simulink subsystem "PvtSubSys_VSM_LCK"  (R2020b)
settings: Solver=VariableStepAuto  StartTime=0.0  StopTime=10.0  RelTol=1e-3
values from neighbouring files (symbols this model uses):
  LCK_STATE : value not decoded    [LCK.sldd]
  P_VSM_LCK_A1 = 15.0    [LCK.sldd]
  P_VSM_LCK_AbsEspInTime = 3.0    [LCK.sldd]
  P_VSM_LCK_absLongitudeAccIn = 2.5    [LCK.sldd]
  P_VSM_LCK_absLongitudeAccOut = 3.0    [LCK.sldd]
  P_VSM_LCK_AccRateIn = 30.0    [LCK.sldd]
  P_VSM_LCK_AccRateInTime = 1.5    [LCK.sldd]
  P_VSM_LCK_AccRateOut = 80.0    [LCK.sldd]
  P_VSM_LCK_AccrPelOut = 30.0    [LCK.sldd]
  P_VSM_LCK_AccrPelRateOut = 0.0    [LCK.sldd]
  P_VSM_LCK_BrakePressIn = 3.0    [LCK.sldd]
  P_VSM_LCK_BrakePressInTime = 1.5    [LCK.sldd]
  P_VSM_LCK_BrakePressOut = 5.0    [LCK.sldd]
  P_VSM_LCK_C0 = 0.4    [LCK.sldd]
  P_VSM_LCK_DrvInputTrqValueIn = 2.0    [LCK.sldd]
  P_VSM_LCK_DrvInputTrqValueInTime = 3.0    [LCK.sldd]
  P_VSM_LCK_DrvInputTrqValueOut = 2.3    [LCK.sldd]
  P_VSM_LCK_dypreFactor = 1.0    [LCK.sldd]
  P_VSM_LCK_IdleInTime = 2.0    [LCK.sldd]
  P_VSM_LCK_LanechangeSwitch = 0.0    [LCK.sldd]
  P_VSM_LCK_LaneDouble = 1.0    [LCK.sldd]
  P_VSM_LCK_Lanewidthswitch = 1.0    [LCK.sldd]
  P_VSM_LCK_LateralAcceIn = 3.0    [LCK.sldd]
  P_VSM_LCK_LateralAcceInTime = 3.0    [LCK.sldd]
  P_VSM_LCK_LateralAcceOut = 3.5    [LCK.sldd]
  P_VSM_LCK_LCDrvInputTrqValueOut = 3.0    [LCK.sldd]
  P_VSM_LCK_LCOverrideTime = 0.6    [LCK.sldd]
  P_VSM_LCK_LCOverrideValue = 1.5    [LCK.sldd]
  P_VSM_LCK_LongitudeAccIn = 3.0    [LCK.sldd]
  P_VSM_LCK_LongitudeAccInTime = 3.0    [LCK.sldd]
  P_VSM_LCK_LongitudeAccOut = 3.5    [LCK.sldd]
  P_VSM_LCK_OverrideInTime = 3.0    [LCK.sldd]
  P_VSM_LCK_OverrideTime = 0.3    [LCK.sldd]
  P_VSM_LCK_OverrideValue = 1.2    [LCK.sldd]
  P_VSM_LCK_ParamA1 : value not decoded    [LCK.sldd]
  P_VSM_LCK_PreTime = 0.2    [LCK.sldd]
  P_VSM_LCK_State_Absesp_enable = 1.0    [LCK.sldd]
  P_VSM_LCK_State_Accpedalrate_enable = 0.0    [LCK.sldd]
  P_VSM_LCK_State_Breakpressure_enable = 1.0    [LCK.sldd]
  P_VSM_LCK_State_DriverInputTrqValue_enable = 1.0    [LCK.sldd]
  P_VSM_LCK_State_Eps_enable = 1.0    [LCK.sldd]
  P_VSM_LCK_State_ESSSts_enable = 1.0    [LCK.sldd]
  P_VSM_LCK_State_GEAR_enable = 1.0    [LCK.sldd]
  P_VSM_LCK_State_Handson_enable = 1.0    [LCK.sldd]
  P_VSM_LCK_State_IdleInTime_enable = 0.0    [LCK.sldd]
  P_VSM_LCK_State_Lane_enable = 1.0    [LCK.sldd]
  P_VSM_LCK_State_LaneChange_enable = 1.0    [LCK.sldd]
  P_VSM_LCK_State_LaneCurve_enable = 0.0    [LCK.sldd]
  P_VSM_LCK_State_LateralAcce_enable = 1.0    [LCK.sldd]
  P_VSM_LCK_State_LongitudeAcc_enable = 1.0    [LCK.sldd]
  P_VSM_LCK_State_LSMLine_enable = 1.0    [LCK.sldd]
  P_VSM_LCK_State_Overide_enable = 1.0    [LCK.sldd]
  P_VSM_LCK_State_Param_LaneCurve : value not decoded    [LCK.sldd]
  P_VSM_LCK_State_Param_LaneCurve_Offset : value not decoded    [LCK.sldd]
  P_VSM_LCK_State_Param_LaneWidth : value not decoded    [LCK.sldd]
  P_VSM_LCK_State_Param_LaneWidth_Offset : value not decoded    [LCK.sldd]
  P_VSM_LCK_State_SteerWheelAngle_enable = 1.0    [LCK.sldd]
  P_VSM_LCK_State_SteerWheelSpd_enable = 1.0    [LCK.sldd]
  P_VSM_LCK_State_TargetLaneIn_enable = 1.0    [LCK.sldd]
  P_VSM_LCK_State_TurnLight_enable = 1.0    [LCK.sldd]
  P_VSM_LCK_State_Vehspeed_enable = 1.0    [LCK.sldd]
  P_VSM_LCK_State_Yawsup_enable = 1.0    [LCK.sldd]
  P_VSM_LCK_SteerAngleSpdIn = 150.0    [LCK.sldd]
  P_VSM_LCK_SteerAngleSpdInTime = 3.0    [LCK.sldd]
  P_VSM_LCK_SteerAngleSpdOut = 200.0    [LCK.sldd]
  P_VSM_LCK_SteerWheelAngleIn = 70.0    [LCK.sldd]
  P_VSM_LCK_SteerWheelAngleInTime = 3.0    [LCK.sldd]
  P_VSM_LCK_SteerWheelAngleOut = 90.0    [LCK.sldd]
  P_VSM_LCK_T0 = 0.75    [LCK.sldd]
  P_VSM_LCK_T1 = 15.0    [LCK.sldd]
  P_VSM_LCK_TargetInSwitch = 0.0    [LCK.sldd]
  P_VSM_LCK_Warnarea1 = -0.55    [LCK.sldd]
  P_VSM_LCK_Warnarea2 = -0.35    [LCK.sldd]
  P_VSM_LCK_YawRateIn = 0.2    [LCK.sldd]
  P_VSM_LCK_YawRateInTime = 1.0    [LCK.sldd]
  P_VSM_LCK_YawRateOut = 0.25    [LCK.sldd]
undefined symbols (not defined in the file or in its folder): P_VSM_LSMC_SampleTime
libraries: simulink x275
(part 3 of 5)

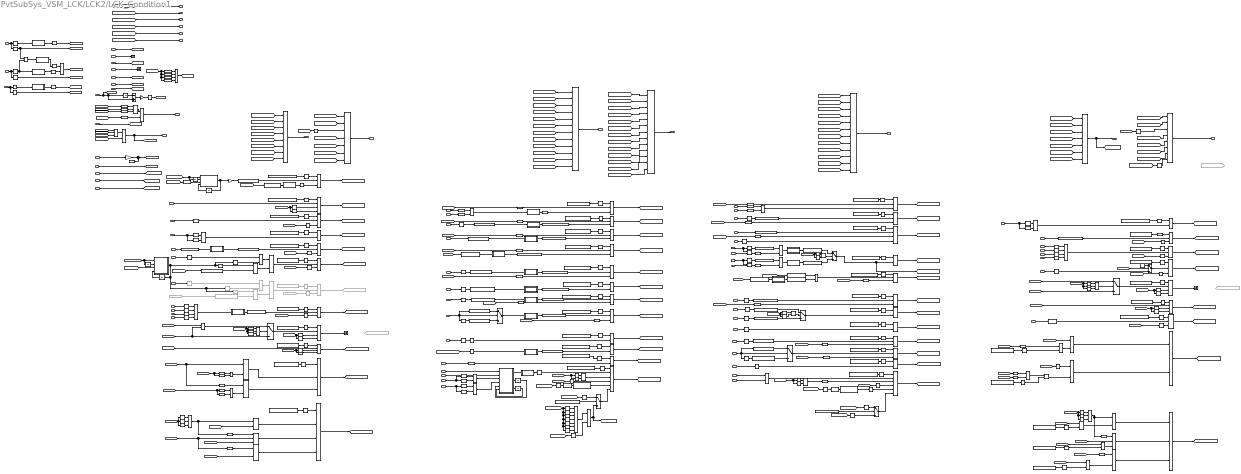
== system PvtSubSys_VSM_LCK/LCK2/LCK_Condition1 ==
  note: 2,3=wrong
  note: Idle2Ready
  note: other2Idle
  note: Active2Ready
  note: Ready2Active
  note: LCK修改记录202010/21
      | 1、去掉TJAlinevalid/LCKlinevalid ;
      |
      |
      |
      |
      | 注：HWAActive=true；将抑制
      | （1）转向灯条件
      | （2）刹车信号；
      | （3）加速踏板信号；
      |
      | 20201102:
      |   TargetP0Exit 换为 TJALineValid
  TJAOn : Inport
  TJASts : Inport  Port=2
  HWAACTIVE : Inport  Port=3
  LCKOn : Inport  Port=4
  VehicleSpd : Inport  Port=5
  VehicleYawRate_rads : Inport  Port=6
  LeftTurnSw : Inport  Port=7
  RightTurnSw : Inport  Port=8
  ECMAccrPellPosnDiagc : Inport  Port=9
  SteerAngleSpd : Inport  Port=10
  ESP_MasterCylindBrakePress : Inport  Port=11
  EPS_DrvInputTrqValue : Inport  Port=12
  EPS_LKATrqOvlDlvdSts : Inport  Port=13
  LKATrqOvlCmdReqValue : Inport  Port=14
  LCKSts : Inport  Port=15
  canESPVDCActive : Inport  Port=16
  canESPPTCActive : Inport  Port=17
  canESPBTCActive : Inport  Port=18
  canABSABSActive : Inport  Port=19
  HandsOffWarnLevel : Inport  Port=20
  canSASSteerWheelAngle : Inport  Port=21
  canABMLateralAcce : Inport  Port=22
  LongitudeAcc : Inport  Port=23
  HandsOn : Inport  Port=24
  TJALineValid : Inport  Port=25
  CURRENT_GEAR : Inport  Port=26
  ESSSts : Inport  Port=27
  LaneCurve : Inport  Port=28
  HWASts : Inport  Port=29
  TJALCKState : Inport  Port=30
  LSSSwtReq : Inport  Port=31
  LeftChange : Inport  Port=32
  RightChange : Inport  Port=33
  FLWhelDy : Inport  Port=34
  FRWhelDy : Inport  Port=35
  LCK_TargetLaneIn : Inport  Port=36
  LCKLineValid : Inport  Port=37
  HWALineValid : Inport  Port=38
  VehConfigLCK : Inport  Port=39
  PLAN_ALC_stsReason : Inport  Port=40
  NOH_Sts : Inport  Port=41
  LSM_PilotRoadSts : Inport  Port=42
  BrkPedalSts : Inport  Port=43
  Abs{,1..10,14..16} (14 alike) : Abs
  Add : Sum  Inputs=-+
  CURRENT_GEAR2 : InportShadow  Port=26
  Compare To Constant : simulink/Logic and Bit Operations/Compare To Constant  relop=<=  const=55  OutDataTypeStr=boolean
  Compare To Constant1 : simulink/Logic and Bit Operations/Compare To Constant  relop=>=  const=P_VSM_LCK_YawRateOut  OutDataTypeStr=boolean
  Compare To Constant10 : simulink/Logic and Bit Operations/Compare To Constant  relop=>  const=0.5  OutDataTypeStr=boolean
  Compare To Constant{100..101,113,125,250} (5 alike) : simulink/Logic and Bit Operations/Compare To Constant  relop===  const=3  OutDataTypeStr=boolean
  Compare To Constant102 : simulink/Logic and Bit Operations/Compare To Constant  relop===  const=2  OutDataTypeStr=boolean
  Compare To Constant103 : simulink/Logic and Bit Operations/Compare To Constant  relop===  const=2  OutDataTypeStr=boolean
  Compare To Constant{2,4..5,14,17,24,33,36,38,48,51,59,63,66,68,70,72,77,81,85,104..105,107,114,116..118,120,124,127..128,157,165,171,173,176,179,181..182,186,188,195..197,199,207,211..212,226..227,229..231,242,245,248} (56 alike) : simulink/Logic and Bit Operations/Compare To Constant  relop===  const=0  OutDataTypeStr=boolean
  Compare To Constant{6,12,15..16,18,20..22,37,39,44,46,56,67,71,74..75,82..83,86,88,90,94,96,106,119,145,166..167,169..170,172,174..175,184,187,193..194,205,208..209,233..234,240,243,246} (46 alike) : simulink/Logic and Bit Operations/Compare To Constant  relop===  const=1  OutDataTypeStr=boolean
  Compare To Constant108 : simulink/Logic and Bit Operations/Compare To Constant  relop=>=  const=3  OutDataTypeStr=boolean
  Compare To Constant109 : simulink/Logic and Bit Operations/Compare To Constant  relop=<=  const=2  OutDataTypeStr=boolean
  Compare To Constant11 : simulink/Logic and Bit Operations/Compare To Constant  relop===  const=8  OutDataTypeStr=boolean
  Compare To Constant110 : simulink/Logic and Bit Operations/Compare To Constant  relop===  const=8  OutDataTypeStr=boolean
  Compare To Constant111 : simulink/Logic and Bit Operations/Compare To Constant  relop===  const=LCK_STATE.LCK_Idle  OutDataTypeStr=boolean
  Compare To Constant112 : simulink/Logic and Bit Operations/Compare To Constant  relop===  const=10  OutDataTypeStr=boolean
  Compare To Constant115 : simulink/Logic and Bit Operations/Compare To Constant  relop===  const=9  OutDataTypeStr=boolean
  Compare To Constant121 : simulink/Logic and Bit Operations/Compare To Constant  relop=<  const=P_VSM_LCK_AccRateIn  OutDataTypeStr=boolean
  Compare To Constant123 : simulink/Logic and Bit Operations/Compare To Constant  relop=<  const=P_VSM_LCK_SteerWheelAngleIn  OutDataTypeStr=boolean
  Compare To Constant126 : simulink/Logic and Bit Operations/Compare To Constant  relop===  const=9  OutDataTypeStr=boolean
  Compare To Constant129 : simulink/Logic and Bit Operations/Compare To Constant  relop=<  const=P_VSM_LCK_LateralAcceIn  OutDataTypeStr=boolean
  Compare To Constant13 : simulink/Logic and Bit Operations/Compare To Constant  relop=<  const=P_VSM_LCK_DrvInputTrqValueIn  OutDataTypeStr=boolean
  Compare To Constant130 : simulink/Logic and Bit Operations/Compare To Constant  relop=<  const=P_VSM_LCK_LongitudeAccIn  OutDataTypeStr=boolean
  Compare To Constant131 : simulink/Logic and Bit Operations/Compare To Constant  relop=<  const=P_VSM_LCK_absLongitudeAccIn  OutDataTypeStr=boolean
  Compare To Constant132 : simulink/Logic and Bit Operations/Compare To Constant  relop===  const=19  OutDataTypeStr=boolean
  Compare To Constant133 : simulink/Logic and Bit Operations/Compare To Constant  relop===  const=20  OutDataTypeStr=boolean
  Compare To Constant134 : simulink/Logic and Bit Operations/Compare To Constant  relop===  const=25  OutDataTypeStr=boolean
  Compare To Constant135 : simulink/Logic and Bit Operations/Compare To Constant  Commented=on  relop===  const=0  OutDataTypeStr=boolean
  Compare To Constant136 : simulink/Logic and Bit Operations/Compare To Constant  relop=>=  const=P_VSM_LCK_AccrPelRateOut  OutDataTypeStr=boolean
  Compare To Constant137 : simulink/Logic and Bit Operations/Compare To Constant  Commented=on  relop===  const=1  OutDataTypeStr=boolean
  Compare To Constant138 : simulink/Logic and Bit Operations/Compare To Constant  Commented=on  relop===  const=0  OutDataTypeStr=boolean
  Compare To Constant{35,41,54,78,80,139,164,177,238,256,258} (11 alike) : simulink/Logic and Bit Operations/Compare To Constant  relop===  const=5  OutDataTypeStr=boolean
  Compare To Constant140 : simulink/Logic and Bit Operations/Compare To Constant  Commented=on  relop===  const=LCK_STATE.LCK_Idle  OutDataTypeStr=boolean
  Compare To Constant141 : simulink/Logic and Bit Operations/Compare To Constant  Commented=on  relop===  const=1  OutDataTypeStr=boolean
  Compare To Constant142 : simulink/Logic and Bit Operations/Compare To Constant  relop===  const=26  OutDataTypeStr=boolean
  Compare To Constant143 : simulink/Logic and Bit Operations/Compare To Constant  relop===  const=30  OutDataTypeStr=boolean
  Compare To Constant144 : simulink/Logic and Bit Operations/Compare To Constant  relop=>=  const=3  OutDataTypeStr=boolean
  Compare To Constant146 : simulink/Logic and Bit Operations/Compare To Constant  relop=<  const=150  OutDataTypeStr=boolean
  Compare To Constant147 : simulink/Logic and Bit Operations/Compare To Constant  relop=>  const=155  OutDataTypeStr=boolean
  Compare To Constant{69,79,150,153,158,163,178,210,239,251,257,259} (12 alike) : simulink/Logic and Bit Operations/Compare To Constant  relop===  const=6  OutDataTypeStr=boolean
  Compare To Constant159 : simulink/Logic and Bit Operations/Compare To Constant  relop=~=  const=5  OutDataTypeStr=boolean
  Compare To Constant160 : simulink/Logic and Bit Operations/Compare To Constant  relop=~=  const=6  OutDataTypeStr=boolean
  Compare To Constant161 : simulink/Logic and Bit Operations/Compare To Constant  relop=~=  const=5  OutDataTypeStr=boolean
  Compare To Constant162 : simulink/Logic and Bit Operations/Compare To Constant  relop=~=  const=6  OutDataTypeStr=boolean
  Compare To Constant19 : simulink/Logic and Bit Operations/Compare To Constant  relop=>=  const=55  OutDataTypeStr=boolean
  Compare To Constant213 : simulink/Logic and Bit Operations/Compare To Constant  relop=<  const=0  OutDataTypeStr=boolean
  Compare To Constant214 : simulink/Logic and Bit Operations/Compare To Constant  relop=>  const=P_VSM_LCK_LCOverrideValue  OutDataTypeStr=boolean
  Compare To Constant228 : simulink/Logic and Bit Operations/Compare To Constant  relop=>=  const=P_VSM_LCK_IdleInTime  OutDataTypeStr=boolean
  Compare To Constant235 : simulink/Logic and Bit Operations/Compare To Constant  Commented=on  relop===  const=1  OutDataTypeStr=boolean
  Compare To Constant237 : simulink/Logic and Bit Operations/Compare To Constant  relop=>  const=P_VSM_LCK_LCOverrideTime  OutDataTypeStr=boolean
  Compare To Constant{8,42,241,244,247} (5 alike) : simulink/Logic and Bit Operations/Compare To Constant  relop=>  const=3  OutDataTypeStr=boolean
  Compare To Constant249 : simulink/Logic and Bit Operations/Compare To Constant  relop=>  const=P_VSM_LCK_LCDrvInputTrqValueOut  OutDataTypeStr=boolean
  Compare To Constant25 : simulink/Logic and Bit Operations/Compare To Constant  relop=<  const=P_VSM_LCK_BrakePressIn  OutDataTypeStr=boolean
  Compare To Constant252 : simulink/Logic and Bit Operations/Compare To Constant  relop===  const=9  OutDataTypeStr=boolean
  Compare To Constant253 : simulink/Logic and Bit Operations/Compare To Constant  relop===  const=10  OutDataTypeStr=boolean
  Compare To Constant27 : simulink/Logic and Bit Operations/Compare To Constant  relop=>  const=P_VSM_LCK_BrakePressOut  OutDataTypeStr=boolean
  Compare To Constant29 : simulink/Logic and Bit Operations/Compare To Constant  relop=<  const=P_VSM_LCK_YawRateIn  OutDataTypeStr=boolean
  Compare To Constant3 : simulink/Logic and Bit Operations/Compare To Constant  relop===  const=8  OutDataTypeStr=boolean
  Compare To Constant34 : simulink/Logic and Bit Operations/Compare To Constant  relop=<  const=0.005  OutDataTypeStr=boolean
  Compare To Constant40 : simulink/Logic and Bit Operations/Compare To Constant  relop=>=  const=P_VSM_LCK_AccrPelOut  OutDataTypeStr=boolean
  Compare To Constant43 : simulink/Logic and Bit Operations/Compare To Constant  relop===  const=LCK_STATE.LCK_Idle  OutDataTypeStr=boolean
  Compare To Constant45 : simulink/Logic and Bit Operations/Compare To Constant  relop=>  const=0.00667  OutDataTypeStr=boolean
  Compare To Constant49 : simulink/Logic and Bit Operations/Compare To Constant  relop=>  const=0.2  OutDataTypeStr=boolean
  Compare To Constant50 : simulink/Logic and Bit Operations/Compare To Constant  relop=>  const=0.2  OutDataTypeStr=boolean
  Compare To Constant53 : simulink/Logic and Bit Operations/Compare To Constant  relop=<  const=0  OutDataTypeStr=boolean
  Compare To Constant55 : simulink/Logic and Bit Operations/Compare To Constant  relop=>  const=P_VSM_LCK_OverrideValue  OutDataTypeStr=boolean
  Compare To Constant57 : simulink/Logic and Bit Operations/Compare To Constant  relop=>  const=0.2  OutDataTypeStr=boolean
  Compare To Constant61 : simulink/Logic and Bit Operations/Compare To Constant  relop=<  const=2  OutDataTypeStr=boolean
  Compare To Constant64 : simulink/Logic and Bit Operations/Compare To Constant  relop=<  const=2  OutDataTypeStr=boolean
  Compare To Constant65 : simulink/Logic and Bit Operations/Compare To Constant  relop=<  const=2  OutDataTypeStr=boolean
  Compare To Constant7 : simulink/Logic and Bit Operations/Compare To Constant  relop=>  const=P_VSM_LCK_OverrideTime  OutDataTypeStr=boolean
  Compare To Constant73 : simulink/Logic and Bit Operations/Compare To Constant  relop===  const=4  OutDataTypeStr=boolean
  Compare To Constant76 : simulink/Logic and Bit Operations/Compare To Constant  relop=>  const=P_VSM_LCK_AbsEspInTime  OutDataTypeStr=boolean
  Compare To Constant84 : simulink/Logic and Bit Operations/Compare To Constant  relop=>  const=P_VSM_LCK_AccRateOut  OutDataTypeStr=boolean
  Compare To Constant87 : simulink/Logic and Bit Operations/Compare To Constant  relop=>  const=P_VSM_LCK_SteerWheelAngleOut  OutDataTypeStr=boolean
  Compare To Constant89 : simulink/Logic and Bit Operations/Compare To Constant  relop=~=  const=4  OutDataTypeStr=boolean
  Compare To Constant91 : simulink/Logic and Bit Operations/Compare To Constant  relop=>  const=P_VSM_LCK_DrvInputTrqValueOut  OutDataTypeStr=boolean
  Compare To Constant92 : simulink/Logic and Bit Operations/Compare To Constant  relop=~=  const=5  OutDataTypeStr=boolean
  Compare To Constant93 : simulink/Logic and Bit Operations/Compare To Constant  relop=>  const=P_VSM_LCK_SteerAngleSpdOut  OutDataTypeStr=boolean
  Compare To Constant95 : simulink/Logic and Bit Operations/Compare To Constant  relop=>  const=1  OutDataTypeStr=boolean
  Compare To Constant97 : simulink/Logic and Bit Operations/Compare To Constant  relop=>  const=P_VSM_LCK_LateralAcceOut  OutDataTypeStr=boolean
  Compare To Constant98 : simulink/Logic and Bit Operations/Compare To Constant  relop=>  const=P_VSM_LCK_LongitudeAccOut  OutDataTypeStr=boolean
  Compare To Constant99 : simulink/Logic and Bit Operations/Compare To Constant  relop=>  const=P_VSM_LCK_absLongitudeAccOut  OutDataTypeStr=boolean
  Compare To Constant122 : simulink/Logic and Bit Operations/Compare To Constant  relop=<  const=P_VSM_LCK_SteerAngleSpdIn  OutDataTypeStr=boolean
  Compare To Constant168 : simulink/Logic and Bit Operations/Compare To Constant  relop=>=  const=155  OutDataTypeStr=boolean
  Compare To Constant183 : simulink/Logic and Bit Operations/Compare To Constant  relop=>=  const=155  OutDataTypeStr=boolean
  Compare To Constant198 : simulink/Logic and Bit Operations/Compare To Constant  relop=<=  const=55  OutDataTypeStr=boolean
  Compare To Constant206 : simulink/Logic and Bit Operations/Compare To Constant  relop=>  const=P_VSM_LCK_OverrideInTime  OutDataTypeStr=boolean
  Compare To Constant23 : simulink/Logic and Bit Operations/Compare To Constant  relop=>  const=P_VSM_LCK_AccRateInTime  OutDataTypeStr=boolean
  Compare To Constant26 : simulink/Logic and Bit Operations/Compare To Constant  relop=>  const=P_VSM_LCK_BrakePressInTime  OutDataTypeStr=boolean
  Compare To Constant28 : simulink/Logic and Bit Operations/Compare To Constant  relop=>  const=P_VSM_LCK_SteerWheelAngleInTime  OutDataTypeStr=boolean
  Compare To Constant30 : simulink/Logic and Bit Operations/Compare To Constant  relop=>  const=P_VSM_LCK_YawRateInTime  OutDataTypeStr=boolean
  Compare To Constant31 : simulink/Logic and Bit Operations/Compare To Constant  relop=>  const=P_VSM_LCK_DrvInputTrqValueInTime  OutDataTypeStr=boolean
  Compare To Constant32 : simulink/Logic and Bit Operations/Compare To Constant  relop=>  const=P_VSM_LCK_LateralAcceInTime  OutDataTypeStr=boolean
  Compare To Constant47 : simulink/Logic and Bit Operations/Compare To Constant  relop=>=  const=0  OutDataTypeStr=boolean
  Compare To Constant52 : simulink/Logic and Bit Operations/Compare To Constant  relop=>=  const=60  OutDataTypeStr=boolean
  Compare To Constant58 : simulink/Logic and Bit Operations/Compare To Constant  relop=>  const=P_VSM_LCK_LongitudeAccInTime  OutDataTypeStr=boolean
  Compare To Constant60 : simulink/Logic and Bit Operations/Compare To Constant  relop=<  const=150  OutDataTypeStr=boolean
  Compare To Constant62 : simulink/Logic and Bit Operations/Compare To Constant  relop=<  const=150  OutDataTypeStr=boolean
  Compare To Constant9 : simulink/Logic and Bit Operations/Compare To Constant  relop=>  const=P_VSM_LCK_SteerAngleSpdInTime  OutDataTypeStr=boolean
  Constant : Constant  Value=1.3
  Constant1 : Constant  Value=0
  Constant2 : Constant  Value=P_VSM_LCK_LanechangeSwitch
  Constant3 : Constant  Value=P_VSM_LCK_LanechangeSwitch
  Data Type Conversion12 : DataTypeConversion  OutDataTypeStr=uint8
  Detect Increase1 : simulink/Logic and Bit Operations/Detect Increase  vinit=0.0  OutDataTypeStr=boolean
  Detect Increase2 : simulink/Logic and Bit Operations/Detect Increase  vinit=0.0  OutDataTypeStr=boolean
  EPS_DrvInputTrqValue{1..4} (4 alike) : InportShadow  Port=12
  EPS_LKATrqOvlDlvdSts1 : InportShadow  Port=13
  ESP_MasterCylindBrakePress1 : InportShadow  Port=11
  ESSSts2 : InportShadow  Port=27
  Enlong3s1 : Subsystem
  Enlong3s3 : Subsystem
  From128 : From  Commented=on  GotoTag=TJA_Active
  From48 : From  Commented=on  GotoTag=Con_TJALane_Ready2Idle
  From80 : From  Commented=on  GotoTag=TJALCKState
  Gain : Gain  Gain=0.02
  Gain1 : Gain  Gain=1.03
  Gain2 : Gain  Gain=50
  Goto20 : Goto  Commented=on  GotoTag=Con_Handson_TJAIdle2Ready
  Goto34 : Goto  Commented=on  GotoTag=Con_Lane_Idle2Ready
  Goto8 : Goto  Commented=on  GotoTag=Con_Lane_Ready2Idle
  HandsOn1 : InportShadow  Port=24
  LKATrqOvlCmdReqValue1 : InportShadow  Port=14
  LaneCurve1 : InportShadow  Port=28
  LeftChange1 : InportShadow  Port=32
  LeftTurnSw1 : InportShadow  Port=7
  Logical Operator{,2..4,14,22,29,57,63,65..66,69,74,76,78,102,118,124,133} (19 alike) : Logic  Operator=OR  AllPortsSameDT=off  OutDataTypeStr=boolean
  Logical Operator1 : Logic  Operator=NOT  AllPortsSameDT=off  OutDataTypeStr=boolean
  Logical Operator{5,7,10,15,19..20,26,30,33,36,38,40,45,49..50,54,56,72,77,80..81,84,87,89,93..94,96,100,105,116..117} (31 alike) : Logic  AllPortsSameDT=off  OutDataTypeStr=boolean
  Logical Operator{6,27,43,86,101,103} (6 alike) : Logic  Operator=OR  Inputs=4  AllPortsSameDT=off  OutDataTypeStr=boolean
  Logical Operator{8,11,37,39,53,58,64,67..68,70..71,75,90,104,107,109..112} (19 alike) : Logic  Operator=OR  Inputs=3  AllPortsSameDT=off  OutDataTypeStr=boolean
  Logical Operator12 : Logic  Inputs=8  AllPortsSameDT=off  OutDataTypeStr=boolean
  Logical Operator{13,44,47..48,51..52,61,79,85,88,92,95,97} (13 alike) : Logic  Inputs=3  AllPortsSameDT=off  OutDataTypeStr=boolean
  Logical Operator132 : Logic  Operator=NOT  AllPortsSameDT=off  OutDataTypeStr=boolean
  Logical Operator16 : Logic  Inputs=13  AllPortsSameDT=off  OutDataTypeStr=boolean
  Logical Operator17 : Logic  Inputs=12  AllPortsSameDT=off  OutDataTypeStr=boolean
  Logical Operator{21,34,62,99} (4 alike) : Logic  Inputs=4  AllPortsSameDT=off  OutDataTypeStr=boolean
  Logical Operator28 : Logic  Operator=OR  Inputs=7  AllPortsSameDT=off  OutDataTypeStr=boolean
  Logical Operator31 : Logic  Operator=OR  Inputs=12  AllPortsSameDT=off  OutDataTypeStr=boolean
  Logical Operator32 : Logic  Inputs=6  AllPortsSameDT=off  OutDataTypeStr=boolean
  Logical Operator35 : Logic  Operator=OR  Inputs=6  AllPortsSameDT=off  OutDataTypeStr=boolean
  Logical Operator46 : Logic  Commented=on  AllPortsSameDT=off  OutDataTypeStr=boolean
  Logical Operator55 : Logic  Commented=on  AllPortsSameDT=off  OutDataTypeStr=boolean
  Logical Operator59 : Logic  Commented=on  Operator=OR  AllPortsSameDT=off  OutDataTypeStr=boolean
  Logical Operator60 : Logic  Commented=on  Operator=OR  Inputs=3  AllPortsSameDT=off  OutDataTypeStr=boolean
  Logical Operator82 : Logic  Inputs=7  AllPortsSameDT=off  OutDataTypeStr=boolean
  Logical Operator83 : Logic  Operator=OR  Inputs=8  AllPortsSameDT=off  OutDataTypeStr=boolean
  Logical Operator9 : Logic  Operator=OR  Inputs=7  AllPortsSameDT=off  OutDataTypeStr=boolean
  LongitudeAcc3 : InportShadow  Port=23
  MATLAB Function : MATLAB Function  TreatAsAtomicUnit=on
  MATLAB Function1 : MATLAB Function  TreatAsAtomicUnit=on
  MATLAB Function3 : MATLAB Function  TreatAsAtomicUnit=on
  NOT : Logic  Operator=NOT  IconShape=distinctive  AllPortsSameDT=off  OutDataTypeStr=boolean
  NOT1 : Logic  Operator=NOT  IconShape=distinctive  AllPortsSameDT=off  OutDataTypeStr=boolean
  NOT2 : Logic  Operator=NOT  IconShape=distinctive  AllPortsSameDT=off  OutDataTypeStr=boolean
  Product : Product
  Product1 : Product
  RightChange1 : InportShadow  Port=33
  RightTurnSw1 : InportShadow  Port=8
  SteerAngleSpd1 : InportShadow  Port=10
  Subsystem1 : Subsystem  mask{Ts=P_VSM_LSMC_SampleTime, Max=10}
      mask prompts: Ts "Sample Time:"; Max "Max Limit:"
      mask Display:
      | Ts=get_param(gcb,'Ts');
      | Max=get_param(gcb,'Max');
      | disp(['Ts:' Ts '\n' 'Max:' Max ]);
  Subsystem10 : Subsystem  mask{Ts=P_VSM_LSMC_SampleTime, Max=10}
      mask prompts: Ts "Sample Time:"; Max "Max Limit:"
      mask Display:
      | Ts=get_param(gcb,'Ts');
      | Max=get_param(gcb,'Max');
      | disp(['Ts:' Ts '\n' 'Max:' Max ]);
  Subsystem11 : Subsystem  mask{Ts=P_VSM_LSMC_SampleTime, Max=10}
      mask prompts: Ts "Sample Time:"; Max "Max Limit:"
      mask Display:
      | Ts=get_param(gcb,'Ts');
      | Max=get_param(gcb,'Max');
      | disp(['Ts:' Ts '\n' 'Max:' Max ]);
  Subsystem12 : Subsystem  mask{Ts=P_VSM_LSMC_SampleTime, Max=10}
      mask prompts: Ts "Sample Time:"; Max "Max Limit:"
      mask Display:
      | Ts=get_param(gcb,'Ts');
      | Max=get_param(gcb,'Max');
      | disp(['Ts:' Ts '\n' 'Max:' Max ]);
  Subsystem13 : Subsystem  mask{Ts=P_VSM_LSMC_SampleTime, Max=10}
      mask prompts: Ts "Sample Time:"; Max "Max Limit:"
      mask Display:
      | Ts=get_param(gcb,'Ts');
      | Max=get_param(gcb,'Max');
      | disp(['Ts:' Ts '\n' 'Max:' Max ]);
  Subsystem14 : Subsystem  mask{Ts=P_VSM_LSMC_SampleTime, Max=10}
      mask prompts: Ts "Sample Time:"; Max "Max Limit:"
      mask Display:
      | Ts=get_param(gcb,'Ts');
      | Max=get_param(gcb,'Max');
      | disp(['Ts:' Ts '\n' 'Max:' Max ]);
  Subsystem15 : Subsystem  mask{Ts=P_VSM_LSMC_SampleTime, Max=10}
      mask prompts: Ts "Sample Time:"; Max "Max Limit:"
      mask Display:
      | Ts=get_param(gcb,'Ts');
      | Max=get_param(gcb,'Max');
      | disp(['Ts:' Ts '\n' 'Max:' Max ]);
  Subsystem16 : Subsystem  mask{Ts=P_VSM_LSMC_SampleTime, Max=10}
      mask prompts: Ts "Sample Time:"; Max "Max Limit:"
      mask Display:
      | Ts=get_param(gcb,'Ts');
      | Max=get_param(gcb,'Max');
      | disp(['Ts:' Ts '\n' 'Max:' Max ]);
  Subsystem17 : Subsystem  mask{Ts=P_VSM_LSMC_SampleTime, Max=10}
      mask prompts: Ts "Sample Time:"; Max "Max Limit:"
      mask Display:
      | Ts=get_param(gcb,'Ts');
      | Max=get_param(gcb,'Max');
      | disp(['Ts:' Ts '\n' 'Max:' Max ]);
  Subsystem18 : Subsystem  mask{Ts=P_VSM_LSMC_SampleTime, Max=10}
      mask prompts: Ts "Sample Time:"; Max "Max Limit:"
      mask Display:
      | Ts=get_param(gcb,'Ts');
      | Max=get_param(gcb,'Max');
      | disp(['Ts:' Ts '\n' 'Max:' Max ]);
  Subsystem19 : Subsystem  mask{Ts=P_VSM_LSMC_SampleTime, Max=10}
      mask prompts: Ts "Sample Time:"; Max "Max Limit:"
      mask Display:
      | Ts=get_param(gcb,'Ts');
      | Max=get_param(gcb,'Max');
      | disp(['Ts:' Ts '\n' 'Max:' Max ]);
  Subsystem2 : Subsystem  mask{Ts=P_VSM_LSMC_SampleTime, Max=10}
      mask prompts: Ts "Sample Time:"; Max "Max Limit:"
      mask Display:
      | Ts=get_param(gcb,'Ts');
      | Max=get_param(gcb,'Max');
      | disp(['Ts:' Ts '\n' 'Max:' Max ]);
  Subsystem20 : Subsystem  mask{Ts=P_VSM_LSMC_SampleTime, Max=10}
      mask prompts: Ts "Sample Time:"; Max "Max Limit:"
      mask Display:
      | Ts=get_param(gcb,'Ts');
      | Max=get_param(gcb,'Max');
      | disp(['Ts:' Ts '\n' 'Max:' Max ]);
  Subsystem21 : Subsystem  mask{Ts=P_VSM_LSMC_SampleTime, Max=10}
      mask prompts: Ts "Sample Time:"; Max "Max Limit:"
      mask Display:
      | Ts=get_param(gcb,'Ts');
      | Max=get_param(gcb,'Max');
      | disp(['Ts:' Ts '\n' 'Max:' Max ]);
  Subsystem3 : Subsystem  mask{Ts=P_VSM_LSMC_SampleTime, Max=10}
      mask prompts: Ts "Sample Time:"; Max "Max Limit:"
      mask Display:
      | Ts=get_param(gcb,'Ts');
      | Max=get_param(gcb,'Max');
      | disp(['Ts:' Ts '\n' 'Max:' Max ]);
  Subsystem4 : Subsystem  mask{Ts=P_VSM_LSMC_SampleTime, Max=10}
      mask prompts: Ts "Sample Time:"; Max "Max Limit:"
      mask Display:
      | Ts=get_param(gcb,'Ts');
      | Max=get_param(gcb,'Max');
      | disp(['Ts:' Ts '\n' 'Max:' Max ]);
  Subsystem5 : Subsystem  mask{Ts=P_VSM_LSMC_SampleTime, Max=10}
      mask prompts: Ts "Sample Time:"; Max "Max Limit:"
      mask Display:
      | Ts=get_param(gcb,'Ts');
      | Max=get_param(gcb,'Max');
      | disp(['Ts:' Ts '\n' 'Max:' Max ]);
  Subsystem7 : Subsystem  mask{Ts=P_VSM_LSMC_SampleTime, Max=10}
      mask prompts: Ts "Sample Time:"; Max "Max Limit:"
      mask Display:
      | Ts=get_param(gcb,'Ts');
      | Max=get_param(gcb,'Max');
      | disp(['Ts:' Ts '\n' 'Max:' Max ]);
  Subsystem8 : Subsystem  mask{Ts=P_VSM_LSMC_SampleTime, Max=10}
      mask prompts: Ts "Sample Time:"; Max "Max Limit:"
      mask Display:
      | Ts=get_param(gcb,'Ts');
      | Max=get_param(gcb,'Max');
      | disp(['Ts:' Ts '\n' 'Max:' Max ]);
  Subsystem9 : Subsystem  mask{Ts=P_VSM_LSMC_SampleTime, Max=10}
      mask prompts: Ts "Sample Time:"; Max "Max Limit:"
      mask Display:
      | Ts=get_param(gcb,'Ts');
      | Max=get_param(gcb,'Max');
      | disp(['Ts:' Ts '\n' 'Max:' Max ]);
  Sum : Sum  Inputs=|++
  Switch{,1..8} (9 alike) : Switch  Criteria=u2 > Threshold
  Terminator{,2..4} (4 alike) : Terminator
  Unit Delay{1..7} (7 alike) : UnitDelay  SampleTime=-1  HasFrameUpgradeWarning=on
  VehicleYawRate_rads1 : InportShadow  Port=6
  canABMLateralAcce3 : InportShadow  Port=22
  canABSABSActive2 : InportShadow  Port=19
  canESPBTCActive2 : InportShadow  Port=18
  canESPPTCActive2 : InportShadow  Port=17
  canESPVDCActive2 : InportShadow  Port=16
  canSASSteerWheelAngle2 : InportShadow  Port=21
  param_1 : Constant  Value=P_VSM_LCK_State_GEAR_enable
  param_10 : Constant  Value=P_VSM_LCK_State_LaneChange_enable
  param_11 : Constant  Value=P_VSM_LCK_State_Accpedalrate_enable
  param_12 : Constant  Value=P_VSM_LCK_State_Overide_enable
  param_13 : Constant  Value=P_VSM_LCK_State_Vehspeed_enable
  param_14 : Constant  Value=P_VSM_LCK_State_Vehspeed_enable
  param_{15,23,26,43} (4 alike) : Constant  Value=P_VSM_LCK_State_Lane_enable
  param_16 : Constant  Value=P_VSM_LCK_State_LaneChange_enable
  param_17 : Constant  Value=P_VSM_LCK_State_LaneCurve_enable
  param_18 : Constant  Value=P_VSM_LCK_State_ESSSts_enable
  param_19 : Constant  Value=P_VSM_LCK_State_Eps_enable
  param_2 : Constant  Value=P_VSM_LCK_State_Absesp_enable
  param_20 : Constant  Value=P_VSM_LCK_State_ESSSts_enable
  param_21 : Constant  Value=P_VSM_LCK_State_LaneCurve_enable
  param_22 : Constant  Commented=on  Value=P_VSM_LCK_State_Handson_enable
  param_24 : Constant  Value=P_VSM_LCK_State_Yawsup_enable
  param_25 : Constant  Value=P_VSM_LCK_State_GEAR_enable
  param_27 : Constant  Value=P_VSM_LCK_State_Absesp_enable
  param_28 : Constant  Value=P_VSM_LCK_State_Handson_enable
  param_29 : Constant  Value=P_VSM_LCK_State_TargetLaneIn_enable
  param_3 : Constant  Value=P_VSM_LCK_State_Handson_enable
  param_{30,32..33,39} (4 alike) : Constant  Value=P_VSM_LCK_State_LSMLine_enable
  param_31 : Constant  Value=P_VSM_LCK_State_Vehspeed_enable
  param_34 : Constant  Value=P_VSM_LCK_State_SteerWheelAngle_enable
  param_35 : Constant  Value=P_VSM_LCK_State_DriverInputTrqValue_enable
  param_36 : Constant  Value=P_VSM_LCK_State_TurnLight_enable
  param_37 : Constant  Value=P_VSM_LCK_State_LateralAcce_enable
  param_38 : Constant  Value=P_VSM_LCK_State_LongitudeAcc_enable
  param_4 : Constant  Value=P_VSM_LCK_State_Eps_enable
  param_40 : Constant  Value=P_VSM_LCK_State_SteerWheelSpd_enable
  param_41 : Constant  Value=P_VSM_LCK_State_Breakpressure_enable
  param_42 : Constant  Value=P_VSM_LCK_State_IdleInTime_enable
  param_46 : Constant  Value=P_VSM_LCK_State_Yawsup_enable
  param_47 : Constant  Value=P_VSM_LCK_State_Overide_enable
  param_49 : Constant  Value=P_VSM_LCK_State_TurnLight_enable
  param_5 : Constant  Value=P_VSM_LCK_State_Accpedalrate_enable
  param_52 : Constant  Value=P_VSM_LCK_State_SteerWheelSpd_enable
  param_53 : Constant  Value=P_VSM_LCK_State_Breakpressure_enable
  param_6 : Constant  Value=P_VSM_LCK_State_SteerWheelAngle_enable
  param_7 : Constant  Value=P_VSM_LCK_State_DriverInputTrqValue_enable
  param_8 : Constant  Value=P_VSM_LCK_State_LateralAcce_enable
  param_9 : Constant  Value=P_VSM_LCK_State_LongitudeAcc_enable
  On : Outport
  Off : Outport  Port=2
  Ready2Active : Outport  Port=3
  Idle2Ready : Outport  Port=4
  Ready2Idle : Outport  Port=5
  Active2Ready : Outport  Port=6
  TJA_Idle2Ready : Outport  Port=7
  TJA_Ready2Idle : Outport  Port=8
  LCK_Con_SteerAngleSpd_ LCKExit : Outport  Port=9
  LCK_Con_BrakePress_ LCKExit : Outport  Port=10
  LCK_Con_OverRide_ LCKExit : Outport  Port=11
  LCK_Con_AccPedalRate_LCKExit : Outport  Port=12
  LCK_Con_SteerWheelAngle_ LCKExit : Outport  Port=13
  LCK_Con_DriverInput_ LCKExit : Outport  Port=14
  LCK_TJAReady2Active : Outport  Port=15
  wires:
  NOT2/1 -> Logical Operator83/8
  [Con_TargetLaneIn_Idle2Ready] -> NOT2/1
  Compare To Constant145/1 -> Logical Operator99/4
  BrkPedalSts/1 -> Compare To Constant145/1
  Enlong3s1/1(Signal_NOH_SysInfoDisplay) -> Logical Operator35/5
  [PLAN_ALC_stsReason] -> Compare To Constant103/1
  Compare To Constant103/1 -> Detect Increase2/1
  Detect Increase2/1 -> Enlong3s1/1(In1)
  NOT/1 -> Logical Operator32/5
  Enlong3s3/1(Signal_NOH_SysInfoDisplay) -> NOT/1
  Detect Increase1/1 -> Enlong3s3/1(In1)
  Compare To Constant102/1 -> Detect Increase1/1
  [PLAN_ALC_stsReason] -> Compare To Constant102/1
  PLAN_ALC_stsReason/1 -> [PLAN_ALC_stsReason]
  Compare To Constant101/1 -> Logical Operator110/3
  Compare To Constant100/1 -> Logical Operator109/1
  Compare To Constant81/1 -> Logical Operator105/2
  [TJA_Active] -> Compare To Constant2/1
  Compare To Constant2/1 -> Logical Operator117/1
  [TJA_Active] -> Logical Operator116/1
  Compare To Constant78/1 -> Switch/3
  [HWA_Sts] -> Compare To Constant35/1, Compare To Constant79/1
  Compare To Constant35/1 -> Logical Operator14/1
  Compare To Constant79/1 -> Logical Operator14/2
  Compare To Constant69/1 -> Logical Operator4/2
  Compare To Constant54/1 -> Logical Operator4/1
  [HWA_Sts] -> Compare To Constant69/1, Compare To Constant54/1
  Compare To Constant51/1 -> Logical Operator54/1
  [TJA_Active] -> Logical Operator7/1, Compare To Constant51/1
  [TJA_Active] -> Compare To Constant81/1
  [TJA_Active] -> Logical Operator/2
  Compare To Constant197/1 -> Logical Operator81/1
  Compare To Constant212/1 -> Logical Operator89/1
  [TJA_Active] -> Compare To Constant212/1
  Compare To Constant259/1 -> Logical Operator110/1
  Compare To Constant258/1 -> Logical Operator110/2
  [HWA_Sts] -> Compare To Constant259/1, Compare To Constant258/1, Compare To Constant101/1
  Logical Operator109/1 -> Logical Operator84/1, Compare To Constant199/1
  Compare To Constant257/1 -> Logical Operator109/3
  Compare To Constant256/1 -> Logical Operator109/2
  [HWA_Sts] -> Compare To Constant256/1, Compare To Constant257/1, Compare To Constant100/1
  HWASts/1 -> [HWA_Sts]
  Logical Operator103/1 -> [TJA_Active]
  [TJA_Sts] -> Compare To Constant250/1, Compare To Constant251/1, Compare To Constant252/1, Compare To Constant253/1
  Compare To Constant253/1 -> Logical Operator103/4
  Compare To Constant252/1 -> Logical Operator103/3
  Compare To Constant251/1 -> Logical Operator103/2
  Compare To Constant250/1 -> Logical Operator103/1
  HWAACTIVE/1 -> Terminator/1
  Compare To Constant248/1 -> [HWALineNotValid]
  Compare To Constant247/1 -> [HWALineValid]
  Subsystem21/1(Out1) -> Compare To Constant247/1
  Compare To Constant246/1 -> Subsystem21/1(In1)
  HWALineValid/1 -> Compare To Constant248/1, Compare To Constant246/1
  TJALineValid/1 -> Compare To Constant243/1, Compare To Constant245/1
  Compare To Constant243/1 -> Logical Operator26/2, Subsystem16/1(In1)
  Subsystem16/1(Out1) -> Compare To Constant244/1
  Compare To Constant244/1 -> Logical Operator76/2
  Compare To Constant245/1 -> [TJALineNotValid]
  Compare To Constant242/1 -> Logical Operator26/1, [LCKLineNotValid]
  Compare To Constant241/1 -> [LCKLineValid]
  Subsystem15/1(Out1) -> Compare To Constant241/1
  Compare To Constant240/1 -> Subsystem15/1(In1)
  LCKLineValid/1 -> Compare To Constant240/1, Compare To Constant242/1
  Logical Operator85/1 -> Logical Operator86/3
  [TJALineValid] -> Logical Operator6/2
  Unit Delay7/1 -> MATLAB Function1/2(HandsOff_Ready2IdleK1)
  Logical Operator61/1 -> Logical Operator/1  "On"
  Logical Operator/1 -> On/1, [LCKOn]
  Compare To Constant77/1 -> Logical Operator53/3
  Compare To Constant157/1 -> Logical Operator53/2
  Compare To Constant104/1 -> Logical Operator53/1
  [VehConfigLCK] -> Compare To Constant104/1
  VehConfigLCK/1 -> [VehConfigLCK]
  [VehConfigLCK] -> Logical Operator61/3
  Unit Delay6/1 -> MATLAB Function3/2(Ready2IdleK1)
  Compare To Constant19/1 -> Logical Operator32/4
  [IP_V_Disp_kmh] -> Compare To Constant19/1
  Compare To Constant/1 -> Logical Operator35/4
  [IP_V_Disp_kmh] -> Compare To Constant/1
  [Con_LaneChange_Active2Ready] -> Logical Operator31/12
  [Con_CURRENT_GEAR_Active2Ready] -> Logical Operator31/11
  [Con_LongitudeAcc_Active2Ready] -> Logical Operator31/10
  [Con_LateralAcc_Active2Ready] -> Logical Operator31/9
  [Con_EpsSta_Active2Ready] -> Logical Operator31/8
  [Con_DriverInput_Active2Ready] -> Logical Operator31/7
  [Con_SteerWheelAngle_Active2Ready] -> Logical Operator31/6
  [Con_AccPedalRate_Active2Ready] -> Logical Operator31/5
  [Con_OverRide_Active2Ready] -> Logical Operator31/4
  [Con_BrakePress_Active2Ready] -> Logical Operator31/3
  [Con_SteerAngleSpd_Active2Ready] -> Logical Operator31/2
  [Con_TurnLight_Active2Ready] -> Logical Operator31/1
  [Con_LaneChange_Ready2Active] -> Logical Operator17/12
  [Con_EpsSts_Ready2Active] -> Logical Operator17/11
  [Con_OverRide_Ready2Active] -> Logical Operator17/10
  [Con_CURRENT_GEAR_Ready2Active] -> Logical Operator17/9
  [Con_LongitudeAcc_Ready2Active] -> Logical Operator17/8
  [Con_LateralAcc_Ready2Active] -> Logical Operator17/7
  [Con_DrvInputTrqValue_Ready2active] -> Logical Operator17/6
  [Con_SteerWheelAngle_Ready2active] -> Logical Operator17/5
  [Con_AccPedalRate_Ready2active] -> Logical Operator17/4
  [Con_BrakePress_Ready2Active] -> Logical Operator17/3
  [Con_SteerAngleSpd_Ready2Active] -> Logical Operator17/2
  [Con_TurnLight_Ready2Active] -> Logical Operator17/1
  [Con_InTime_Idle2Ready] -> Logical Operator12/6
  Compare To Constant229/1 -> Logical Operator75/1
  param_42/1 -> Compare To Constant229/1
  Logical Operator75/1 -> [Con_InTime_Idle2Ready]  "VSM_LCK_Con_InTime_Idle2Ready"
  Data Type Conversion12/1 -> MATLAB Function3/3(LCKSts)
  [LCK_Sts] -> Data Type Conversion12/1
  Compare To Constant228/1 -> Logical Operator75/2
  Gain/1 -> Compare To Constant228/1
  Unit Delay5/1 -> MATLAB Function3/4(CountK1)
  MATLAB Function3/1(Count) -> Unit Delay5/1, Gain/1
  [VSM_LCK_Ready2Idle] -> MATLAB Function3/1(Ready2Idle), Unit Delay6/1
  [Con_TargetLaneIn_Idle2Ready] -> Logical Operator82/7
  [Con_LSMLine_Ready2Idle] -> Logical Operator28/4
  [TJA_Active] -> Logical Operator88/2
  [LCKLineNotValid] -> Logical Operator93/1
  [TJALineNotValid] -> Logical Operator94/1
  [HWALineNotValid] -> Logical Operator96/1
  Compare To Constant205/1 -> Logical Operator93/2
  Logical Operator89/1 -> Logical Operator90/3
  Compare To Constant208/1 -> Logical Operator94/2
  param_32/1 -> Compare To Constant205/1
  param_39/1 -> Compare To Constant209/1
  Compare To Constant211/1 -> Logical Operator88/1
  Logical Operator93/1 -> Logical Operator89/2
  Logical Operator90/1 -> [Con_LSMLine_Ready2Idle]  "VSM_LCK_Con_LSMLine_Ready2Idle"
  Logical Operator94/1 -> Logical Operator88/3
  Compare To Constant209/1 -> Logical Operator96/2
  Logical Operator87/1 -> Logical Operator90/1
  Logical Operator88/1 -> Logical Operator90/2
  Logical Operator110/1 -> Logical Operator87/1, Compare To Constant211/1
  Logical Operator96/1 -> Logical Operator87/2
  param_33/1 -> Compare To Constant208/1
  [TJA_Active] -> Logical Operator85/2, Compare To Constant197/1
  [LCKLineValid] -> Logical Operator81/2
  [TJALineValid] -> Logical Operator85/3
  [HWALineValid] -> Logical Operator84/2
  param_30/1 -> Compare To Constant196/1
  Compare To Constant199/1 -> Logical Operator85/1
  Logical Operator86/1 -> [Con_LSMLine_Idle2Ready]  "VSM_LCK_Con_LSMLine_Idle2Ready"
  Logical Operator84/1 -> Logical Operator86/2
  Logical Operator81/1 -> Logical Operator86/4
  Compare To Constant196/1 -> Logical Operator86/1
  Compare To Constant184/1 -> Logical Operator71/3
  [TJA_Active] -> Compare To Constant184/1
  Compare To Constant181/1 -> Logical Operator52/3
  [TJA_Active] -> Compare To Constant181/1
  Compare To Constant46/1 -> Logical Operator11/3
  [TJA_Active] -> Compare To Constant46/1
  Compare To Constant171/1 -> Logical Operator44/3
  [TJA_Active] -> Compare To Constant171/1
  Compare To Constant166/1 -> Logical Operator64/3
  [TJA_Active] -> Compare To Constant166/1
  Compare To Constant178/1 -> Logical Operator27/4
  Compare To Constant177/1 -> Logical Operator27/3
  [HWA_Sts] -> Compare To Constant177/1, Compare To Constant178/1
  Logical Operator27/1 -> [Con_TargetLaneIn_Idle2Ready]  "VSM_LCK_Con_TargetLaneIn_Idle2Ready"
  Compare To Constant165/1 -> Logical Operator27/1
  param_29/1 -> Compare To Constant165/1
  LCK_TargetLaneIn/1 -> Logical Operator27/2
  [HWA_Sts] -> Compare To Constant164/1, Compare To Constant163/1
  Compare To Constant164/1 -> Logical Operator6/3
  Compare To Constant163/1 -> Logical Operator6/4
  [HWA_Sts] -> Compare To Constant162/1, Compare To Constant161/1
  Compare To Constant161/1 -> Logical Operator21/3
  Compare To Constant162/1 -> Logical Operator21/4
  Compare To Constant160/1 -> Logical Operator34/4
  Compare To Constant159/1 -> Logical Operator34/3
  [HWA_Sts] -> Compare To Constant159/1, Compare To Constant160/1
  Compare To Constant158/1 -> Logical Operator101/4
  Compare To Constant41/1 -> Logical Operator101/3
  [HWA_Sts] -> Compare To Constant41/1, Compare To Constant158/1
  [LCK_Sts] -> MATLAB Function1/3(LCKSts)
  [Con_HandOff_Ready2Idle] -> MATLAB Function1/1(HandsOff_Ready2Idle), Unit Delay7/1
  Unit Delay4/1 -> MATLAB Function1/4(yK1)
  Logical Operator53/1 -> Logical Operator105/1
  [LSSSwtReq] -> Compare To Constant157/1
  Logical Operator105/1 -> Off/1  "Off"
  [TJALineNotValid] -> Switch5/1
  [TJALineNotValid] -> Logical Operator21/2
  [TJALineValid] -> Logical Operator74/1
  Logical Operator21/1 -> [Con_TJALane_Ready2Idle]  "VSM_LCK_Con_TJALane_Ready2Idle"
  Compare To Constant21/1 -> Logical Operator21/1
  param_23/1 -> Compare To Constant21/1
  Logical Operator6/1 -> [Con_TJALane_Idle2Ready]  "VSM_LCK_Con_TJALane_Idle2Ready"
  Compare To Constant63/1 -> Logical Operator6/1
  param_15/1 -> Compare To Constant63/1
  Compare To Constant59/1 -> Logical Operator32/3
  Logical Operator14/1 -> Compare To Constant59/1
  Logical Operator4/1 -> Logical Operator35/3
  Switch/1 -> Logical Operator79/2
  [Con_ESSSts_Idle2Ready] -> Logical Operator12/1
  ESSSts/1 -> Compare To Constant92/1, Compare To Constant89/1
  param_20/1 -> Compare To Constant85/1
  Compare To Constant85/1 -> Logical Operator66/1
  Logical Operator66/1 -> [Con_ESSSts_Idle2Ready]  "VSM_LCK_Con_ESSSts_Idle2Ready"
  Compare To Constant92/1 -> Logical Operator72/2
  Logical Operator72/1 -> Logical Operator66/2
  Compare To Constant89/1 -> Logical Operator72/1
  [Con_ESSSts_Ready2Idle] -> Logical Operator28/1
  Compare To Constant72/1 -> Logical Operator63/1
  param_18/1 -> Compare To Constant72/1
  Compare To Constant80/1 -> Logical Operator65/2
  ESSSts2/1 -> Compare To Constant80/1, Compare To Constant73/1
  Logical Operator63/1 -> [Con_ESSSts_Ready2Idle]  "VSM_LCK_Con_ESSSts_Ready2Idle"
  Logical Operator65/1 -> Logical Operator63/2
  Compare To Constant73/1 -> Logical Operator65/1
  Logical Operator22/1 -> Logical Operator32/2
  Compare To Constant49/1 -> Logical Operator35/2
  Compare To Constant65/1 -> Logical Operator36/2
  Subsystem1/1(Out1) -> Compare To Constant49/1
  MATLAB Function/1(y) -> Subsystem1/1(In1)
  Logical Operator45/1 -> MATLAB Function/3(Ldy)
  FRWhelDy/1 -> Compare To Constant57/1, Compare To Constant65/1
  Logical Operator35/1 -> [Con_LaneChange_Ready2Active]  "VSM_LCK_Con_LaneChange_Ready2Active"
  FLWhelDy/1 -> Compare To Constant50/1, Compare To Constant64/1
  Compare To Constant38/1 -> Logical Operator35/1
  param_16/1 -> Compare To Constant38/1
  RightChange1/1 -> MATLAB Function/2(RightChangefg)
  LeftChange1/1 -> MATLAB Function/1(LeftChangefg)
  Unit Delay3/1 -> MATLAB Function/6(Rfgk1)
  MATLAB Function/3(Rfg) -> Unit Delay3/1
  Unit Delay2/1 -> MATLAB Function/5(Lfgk1)
  Compare To Constant57/1 -> Logical Operator36/1
  MATLAB Function/2(Lfg) -> Unit Delay2/1
  Compare To Constant64/1 -> Logical Operator45/2
  Compare To Constant50/1 -> Logical Operator45/1
  Logical Operator36/1 -> MATLAB Function/4(Rdy)
  LeftChange/1 -> Logical Operator22/1
  RightChange/1 -> Logical Operator22/2
  Logical Operator32/1 -> [Con_LaneChange_Active2Ready]  "VSM_LCK_Con_LaneChange_Active2Ready"
  Compare To Constant37/1 -> Logical Operator32/1
  param_10/1 -> Compare To Constant37/1
  [LCK_Sts] -> Compare To Constant111/1
  Subsystem5/1(Out1) -> Compare To Constant7/1
  Logical Operator33/1 -> Subsystem5/1(In1)
  param_14/1 -> Compare To Constant39/1
  Compare To Constant39/1 -> Logical Operator20/2
  Logical Operator20/1 -> Logical Operator116/2
  Compare To Constant18/1 -> Logical Operator19/2
  Logical Operator19/1 -> Logical Operator117/2
  param_13/1 -> Compare To Constant18/1
  param_12/1 -> Compare To Constant175/1
  param_31/1 -> Compare To Constant36/1
  Compare To Constant36/1 -> Logical Operator8/1
  [LCKLineNotValid] -> Switch5/3
  [AccrPellRate] -> Compare To Constant121/1
  Abs3/1 -> [AccrPellRate]
  ECMAccrPellPosnDiagc/1 -> [AccrPel], Unit Delay1/1, Add/2
  Add/1 -> Gain2/1
  Gain2/1 -> Abs3/1
  Unit Delay1/1 -> Add/1
  Logical Operator40/1 -> Logical Operator54/2
  Logical Operator7/1 -> Logical Operator8/2
  Compare To Constant52/1 -> Logical Operator40/1
  Logical Operator54/1 -> Logical Operator8/3
  Compare To Constant60/1 -> Logical Operator40/2
  Logical Operator8/1 -> [Con_VehicleSpd_Idle2Ready]  "VSM_LCK_Con_VehicleSpd_Idle2Ready"
  [IP_V_Disp_kmh] -> Compare To Constant47/1, Compare To Constant62/1
  [IP_V_Disp_kmh] -> Compare To Constant52/1, Compare To Constant60/1
  Compare To Constant116/1 -> Logical Operator62/4
  Compare To Constant20/1 -> Logical Operator5/2
  Logical Operator5/1 -> Logical Operator57/1
  EPS_DrvInputTrqValue/1 -> Product/1, Abs1/1
  VehicleYawRate_rads/1 -> Compare To Constant29/1
  VehicleSpd/1 -> Gain1/1
  LKATrqOvlCmdReqValue/1 -> Product/2  "Override"
  Compare To Constant53/1 -> Logical Operator33/2
  Logical Operator12/1 -> Idle2Ready/1  "VSM_LCK_Idle2Ready"
  Compare To Constant15/1 -> Logical Operator3/1
  Constant/1 -> Sum/2
  Compare To Constant16/1 -> Logical Operator3/2
  TJAOn/1 -> Terminator3/1
  LeftTurnSw/1 -> Compare To Constant15/1
  Abs/1 -> Compare To Constant93/1
  Gain1/1 -> Sum/1
  Product/1 -> Compare To Constant53/1
  Subsystem17/1(Out1) -> Compare To Constant30/1
  EPS_LKATrqOvlDlvdSts/1 -> Compare To Constant61/1
  ESP_MasterCylindBrakePress/1 -> Compare To Constant25/1
  Abs1/1 -> Compare To Constant55/1
  VehicleYawRate_rads1/1 -> Compare To Constant1/1
  Compare To Constant70/1 -> Logical Operator38/2
  ESP_MasterCylindBrakePress1/1 -> Compare To Constant27/1
  RightTurnSw/1 -> Compare To Constant16/1
  TJASts/1 -> [TJA_Sts]
  Logical Operator28/1 -> Ready2Idle/1, [VSM_LCK_Ready2Idle]  "VSM_LCK_Ready2Idle"
  LeftTurnSw1/1 -> Compare To Constant66/1
  RightTurnSw1/1 -> Compare To Constant70/1
  Compare To Constant71/1 -> Logical Operator107/2
  Compare To Constant66/1 -> Logical Operator38/1
  [TJA_Active] -> Compare To Constant71/1
  Abs2/1 -> Compare To Constant122/1
  SteerAngleSpd/1 -> Abs/1
  LCKSts/1 -> [LCK_Sts]
  Compare To Constant17/1 -> Logical Operator95/2
  LCKOn/1 -> [LCK_On]
  Logical Operator31/1 -> Active2Ready/1  "VSM_LCK_Active2Ready"
  Sum/1 -> [IP_V_Disp_kmh]
  canESPBTCActive/1 -> Compare To Constant88/1
  Logical Operator43/1 -> Logical Operator44/2  "absespsup"
  canABSABSActive/1 -> Compare To Constant74/1
  canESPVDCActive/1 -> Compare To Constant75/1
  Compare To Constant74/1 -> Logical Operator43/4
  Compare To Constant119/1 -> Logical Operator44/1
  Compare To Constant82/1 -> Logical Operator43/2
  param_27/1 -> Compare To Constant119/1
  canESPPTCActive/1 -> Compare To Constant82/1
  Logical Operator44/1 -> [Con_AbsEsp_Ready2Idle]  "VSM_LCK_Con_AbsEsp_Ready2Idle"
  Compare To Constant88/1 -> Logical Operator43/3
  Compare To Constant75/1 -> Logical Operator43/1
  HandsOffWarnLevel/1 -> Compare To Constant78/1
  [AccrPellRate] -> Compare To Constant84/1
  param_11/1 -> Compare To Constant83/1
  Compare To Constant83/1 -> Logical Operator47/1
  Logical Operator47/1 -> [Con_AccPedalRate_Active2Ready]  "VSM_LCK_Con_AccPedalRate_Active2Ready"
  Abs8/1 -> Compare To Constant87/1
  Compare To Constant86/1 -> Logical Operator48/1
  canSASSteerWheelAngle/1 -> Abs8/1
  Logical Operator48/1 -> [Con_SteerWheelAngle_Active2Ready]  "VSM_LCK_Con_SteerWheelAngle_Active2Ready"
  param_34/1 -> Compare To Constant86/1
  Compare To Constant87/1 -> Logical Operator48/2
  Abs14/1 -> Compare To Constant91/1
  param_35/1 -> Compare To Constant90/1
  Compare To Constant90/1 -> Logical Operator49/1
  Logical Operator49/1 -> [Con_DriverInput_Active2Ready]  "VSM_LCK_Con_DriverInput_Active2Ready"
  EPS_DrvInputTrqValue2/1 -> Abs14/1
  Compare To Constant94/1 -> Logical Operator50/1
  Compare To Constant95/1 -> Logical Operator50/2
  Logical Operator50/1 -> [Con_EpsSta_Active2Ready]  "VSM_LCK_Con_EpsSta_Active2Ready"
  param_19/1 -> Compare To Constant94/1
  EPS_LKATrqOvlDlvdSts1/1 -> Compare To Constant95/1
  Compare To Constant97/1 -> Logical Operator52/2
  Compare To Constant98/1 -> Switch4/1
  Switch4/1 -> Logical Operator51/2
  LongitudeAcc/1 -> Abs15/1, Switch4/2, Compare To Constant98/1
  Compare To Constant99/1 -> Switch4/3
  Logical Operator51/1 -> [Con_LongitudeAcc_Active2Ready]  "VSM_LCK_Con_LongitudeAcc_Active2Ready"
  Abs16/1 -> Compare To Constant97/1
  canABMLateralAcce/1 -> Abs16/1
  Logical Operator52/1 -> [Con_LateralAcc_Active2Ready]  "VSM_LCK_Con_LateralAcc_Active2Ready"
  Compare To Constant96/1 -> Logical Operator52/1
  param_37/1 -> Compare To Constant96/1
  param_38/1 -> Compare To Constant22/1
  Abs15/1 -> Compare To Constant99/1
  Compare To Constant22/1 -> Logical Operator51/1
  Compare To Constant105/1 -> Logical Operator58/1
  Logical Operator57/1 -> Logical Operator58/2
  HandsOn/1 -> Compare To Constant106/1
  param_3/1 -> Compare To Constant105/1
  Logical Operator58/1 -> [Con_Handson_Idle2Ready]  "VSM_LCK_Con_Handson_Idle2Ready"
  Compare To Constant117/1 -> Logical Operator62/1
  Compare To Constant120/1 -> Logical Operator62/3
  Logical Operator64/1 -> [Con_AbsEsp_Idle2ready]  "VSM_LCK_Con_AbsEsp_Idle2Ready"
  canESPPTCActive2/1 -> Compare To Constant118/1
  param_2/1 -> Compare To Constant114/1
  Compare To Constant118/1 -> Logical Operator62/2
  Compare To Constant114/1 -> Logical Operator64/1
  canESPVDCActive2/1 -> Compare To Constant117/1
  canABSABSActive2/1 -> Compare To Constant116/1
  canESPBTCActive2/1 -> Compare To Constant120/1
  Compare To Constant76/1 -> Logical Operator64/2
  Logical Operator67/1 -> [Con_AccPedalRate_Ready2active]  "VSM_LCK_Con_AccPedalRate_Ready2Active"
  Compare To Constant14/1 -> Logical Operator67/1
  param_5/1 -> Compare To Constant14/1
  canSASSteerWheelAngle2/1 -> Abs4/1
  param_6/1 -> Compare To Constant24/1
  Abs4/1 -> Compare To Constant123/1
  Compare To Constant24/1 -> Logical Operator68/1
  Logical Operator68/1 -> [Con_SteerWheelAngle_Ready2active]  "VSM_LCK_Con_SteerWheelAngle_Ready2Active"
  Logical Operator69/1 -> [Con_DrvInputTrqValue_Ready2active]  "VSM_LCK_Con_DrvInputTrqValue_Ready2Active"
  Compare To Constant124/1 -> Logical Operator69/1
  Abs5/1 -> Compare To Constant13/1
  param_7/1 -> Compare To Constant124/1
  EPS_DrvInputTrqValue3/1 -> Abs5/1
  Compare To Constant131/1 -> Switch1/3
  Logical Operator70/1 -> [Con_LongitudeAcc_Ready2Active]  "VSM_LCK_Con_LongitudeAcc_Ready2Active"
  Abs7/1 -> Compare To Constant129/1
  param_8/1 -> Compare To Constant128/1
  Abs6/1 -> Compare To Constant131/1
  param_9/1 -> Compare To Constant127/1
  Compare To Constant127/1 -> Logical Operator70/1
  LongitudeAcc3/1 -> Compare To Constant130/1, Switch1/2, Abs6/1
  Compare To Constant128/1 -> Logical Operator71/1
  Compare To Constant130/1 -> Switch1/1
  canABMLateralAcce3/1 -> Abs7/1
  Logical Operator71/1 -> [Con_LateralAcc_Ready2Active]  "VSM_LCK_Con_LateralAcc_Ready2Active"
  Logical Operator37/1 -> Switch6/2
  Logical Operator74/1 -> Switch6/1
  [LCKLineValid] -> Switch6/3, Logical Operator74/2
  Logical Operator79/1 -> [Con_HandOff_Ready2Idle]  "VSM_LCK_Con_HandsOff_Ready2Idle"
  Compare To Constant29/1 -> Subsystem17/1(In1)
  Compare To Constant25/1 -> Subsystem20/1(In1)
  Subsystem20/1(Out1) -> Compare To Constant26/1
  Compare To Constant1/1 -> Logical Operator92/2
  Logical Operator92/1 -> [Con_YawRate_Ready2Idle]  "VSM_LCK_Con_YawRate_Ready2Idle"
  Compare To Constant167/1 -> Logical Operator92/1
  param_24/1 -> Compare To Constant167/1
  param_28/1 -> Compare To Constant170/1
  param_26/1 -> Compare To Constant56/1
  Compare To Constant56/1 -> Logical Operator34/1
  Switch5/1 -> Logical Operator34/2
  Logical Operator34/1 -> Terminator2/1  "VSM_LCK_Con_Lane_Ready2Idle"
  Compare To Constant169/1 -> Logical Operator95/1
  param_36/1 -> Compare To Constant169/1
  Logical Operator3/1 -> Logical Operator95/3
  Logical Operator95/1 -> [Con_TurnLight_Active2Ready]  "VSM_LCK_Con_TurnLight_Active2Ready"
  Compare To Constant172/1 -> Logical Operator97/1
  param_40/1 -> Compare To Constant172/1
  Compare To Constant93/1 -> Logical Operator97/2
  Logical Operator97/1 -> [Con_SteerAngleSpd_Active2Ready]  "VSM_LCK_Con_SteerAngleSpd_Active2Ready"
  [TJA_Active] -> Compare To Constant173/1
  Compare To Constant173/1 -> Logical Operator99/3
  param_41/1 -> Compare To Constant174/1
  Compare To Constant174/1 -> Logical Operator99/1
  Compare To Constant27/1 -> Logical Operator99/2
  Logical Operator99/1 -> [Con_BrakePress_Active2Ready]  "VSM_LCK_Con_BrakePress_Active2Ready"
  Compare To Constant175/1 -> Logical Operator100/1
  Logical Operator100/1 -> [Con_OverRide_Active2Ready]  "VSM_LCK_Con_OverRide_Active2Ready"
  param_43/1 -> Compare To Constant176/1
  Compare To Constant176/1 -> Logical Operator101/1
  Switch6/1 -> Logical Operator101/2
  Logical Operator101/1 -> Terminator4/1  "VSM_LCK_Con_Lane_Idle2Ready"
  param_46/1 -> Compare To Constant179/1
  Compare To Constant179/1 -> Logical Operator104/1
  Compare To Constant30/1 -> Logical Operator104/2
  Logical Operator104/1 -> [Con_YawRate_Idle2Ready]  "VSM_LCK_Con_YawRate_Idle2Ready"
  Compare To Constant182/1 -> Logical Operator107/1
  param_49/1 -> Compare To Constant182/1
  Compare To Constant8/1 -> Logical Operator107/3
  Logical Operator107/1 -> [Con_TurnLight_Ready2Active]  "VSM_LCK_Con_TurnLight_Ready2Active"
  param_52/1 -> Compare To Constant186/1
  Compare To Constant186/1 -> Logical Operator111/1
  Logical Operator111/1 -> [Con_SteerAngleSpd_Ready2Active]  "VSM_LCK_Con_SteerAngleSpd_Ready2Active"
  [TJA_Active] -> Compare To Constant187/1
  param_53/1 -> Compare To Constant188/1
  Compare To Constant188/1 -> Logical Operator112/1
  Logical Operator112/1 -> [Con_BrakePress_Ready2Active]  "VSM_LCK_Con_BrakePress_Ready2Active"
  Logical Operator17/1 -> Ready2Active/1  "VSM_LCK_Ready2Active"
  CURRENT_GEAR/1 -> Compare To Constant3/1
  param_25/1 -> Compare To Constant4/1
  Logical Operator2/1 -> [Con_CURRENT_GEAR_Ready2Active]  "VSM_LCK_Con_CURRENT_GEAR_Ready2Active"
  Logical Operator1/1 -> Logical Operator2/2
  Compare To Constant3/1 -> Logical Operator1/1
  Compare To Constant4/1 -> Logical Operator2/1
  [TJA_Active] -> Compare To Constant5/1
  Compare To Constant5/1 -> Logical Operator47/3
  Compare To Constant187/1 -> Logical Operator112/2
  Compare To Constant26/1 -> Logical Operator112/3
  [TJA_Active] -> Compare To Constant6/1
  Compare To Constant6/1 -> Logical Operator67/2
  Compare To Constant23/1 -> Logical Operator67/3
  Compare To Constant55/1 -> Logical Operator33/1
  Subsystem7/1(Out1) -> Compare To Constant8/1
  Logical Operator38/1 -> Subsystem7/1(In1)
  SteerAngleSpd1/1 -> Abs2/1
  Subsystem8/1(Out1) -> Compare To Constant9/1
  Compare To Constant122/1 -> Subsystem8/1(In1)
  Compare To Constant9/1 -> Logical Operator111/3
  Subsystem9/1(Out1) -> Compare To Constant23/1
  Compare To Constant121/1 -> Subsystem9/1(In1)
  Compare To Constant123/1 -> Subsystem11/1(In1)
  Subsystem11/1(Out1) -> Compare To Constant28/1
  Compare To Constant28/1 -> Logical Operator68/2
  Subsystem12/1(Out1) -> Compare To Constant31/1
  Compare To Constant31/1 -> Logical Operator69/2
  Compare To Constant129/1 -> Subsystem13/1(In1)
  Subsystem13/1(Out1) -> Compare To Constant32/1
  Compare To Constant32/1 -> Logical Operator71/2
  Subsystem14/1(Out1) -> Compare To Constant58/1
  Switch1/1 -> Subsystem14/1(In1)
  Compare To Constant58/1 -> Logical Operator70/2
  Subsystem18/1(Out1) -> Compare To Constant76/1
  Logical Operator62/1 -> Subsystem18/1(In1)
  [LCK_On] -> Compare To Constant77/1
  Logical Operator117/1 -> Logical Operator118/2
  Logical Operator116/1 -> Logical Operator118/1
  [IP_V_Disp_kmh] -> Compare To Constant168/1
  [IP_V_Disp_kmh] -> Compare To Constant183/1
  [IP_V_Disp_kmh] -> Compare To Constant198/1
  Compare To Constant168/1 -> Logical Operator124/1
  Compare To Constant198/1 -> Logical Operator124/2
  Logical Operator124/1 -> Logical Operator19/1
  [OverRide] -> Logical Operator132/1
  Logical Operator132/1 -> Subsystem19/1(In1)
  Subsystem19/1(Out1) -> Compare To Constant206/1
  Compare To Constant206/1 -> Logical Operator133/2
  param_47/1 -> Compare To Constant207/1
  Compare To Constant207/1 -> Logical Operator133/1
  Logical Operator133/1 -> [Con_OverRide_Ready2Active]  "VSM_LCK_Con_OverRide_Ready2Active"
  Logical Operator118/1 -> [Con_VehicleSpd_Ready2Idle]  "VSM_LCK_Con_VehicleSpd_Ready2Idle"
  [Con_YawRate_Ready2Idle] -> Logical Operator28/2
  [Con_AbsEsp_Ready2Idle] -> Logical Operator28/6
  [Con_HandOff_Ready2Idle] -> Logical Operator28/5
  [Con_VehicleSpd_Ready2Idle] -> Logical Operator28/3
  CURRENT_GEAR2/1 -> Compare To Constant11/1
  Compare To Constant12/1 -> Logical Operator30/1
  Logical Operator30/1 -> [Con_CURRENT_GEAR_Active2Ready]  "VSM_LCK_Con_CURRENT_GEAR_Active2Ready"
  param_1/1 -> Compare To Constant12/1
  Compare To Constant11/1 -> Logical Operator30/2
  Compare To Constant48/1 -> Logical Operator29/1
  param_4/1 -> Compare To Constant48/1
  Compare To Constant61/1 -> Logical Operator29/2
  Logical Operator29/1 -> [Con_EpsSts_Ready2Active]  "VSM_LCK_Con_EpsSts_Ready2Active"
  Logical Operator56/1 -> Logical Operator57/2
  Compare To Constant106/1 -> Logical Operator5/1
  Compare To Constant107/1 -> Logical Operator56/1
  Compare To Constant111/1 -> Logical Operator56/2
  [Con_AbsEsp_Idle2ready] -> Logical Operator12/5
  [Con_VehicleSpd_Idle2Ready] -> Logical Operator12/3
  [Con_YawRate_Idle2Ready] -> Logical Operator12/2
  [Con_Handson_Idle2Ready] -> Logical Operator12/4
  Compare To Constant170/1 -> Logical Operator79/1
  Logical Operator39/1 -> Switch5/2
  [TJA_Active] -> Compare To Constant17/1
  Compare To Constant33/1 -> Logical Operator11/1
  Logical Operator11/1 -> [Con_LaneCurve_Idle2Ready]  "VSM_LCK_Con_LaneCurve_Idle2Ready"
  LaneCurve/1 -> Compare To Constant34/1
  Compare To Constant34/1 -> Logical Operator11/2
  param_17/1 -> Compare To Constant33/1
  param_21/1 -> Compare To Constant44/1
  Compare To Constant45/1 -> Logical Operator13/2
  Compare To Constant44/1 -> Logical Operator13/1
  LaneCurve1/1 -> Compare To Constant45/1
  Logical Operator13/1 -> [Con_LaneCurve_Ready2Idle]  "VSM_LCK_Con_LaneCurve_Ready2Idle"
  [Con_LaneCurve_Ready2Idle] -> Logical Operator28/7
  [Con_LaneCurve_Idle2Ready] -> Logical Operator12/7
  Compare To Constant183/1 -> Logical Operator20/1
  Compare To Constant47/1 -> Logical Operator15/2
  Compare To Constant62/1 -> Logical Operator15/1
  Logical Operator15/1 -> Logical Operator7/2
  [TJA_Active] -> Compare To Constant68/1
  Compare To Constant68/1 -> Logical Operator13/3
  [Con_AbsEsp_Idle2ready] -> Logical Operator82/4
  [Con_YawRate_Idle2Ready] -> Logical Operator82/2
  [IP_V_Disp_kmh] -> Compare To Constant146/1
  Compare To Constant146/1 -> Logical Operator82/3  "VSM_LCK_Con_TJAVehicleSpd_Idle2Ready"
  Logical Operator82/1 -> TJA_Idle2Ready/1  "VSM_LCK_TJAIdle2Ready"
  [Con_ESSSts_Idle2Ready] -> Logical Operator82/1
  [Con_LaneCurve_Idle2Ready] -> Logical Operator82/6
  [Con_TJALane_Idle2Ready] -> Logical Operator82/5
  [Con_ESSSts_Ready2Idle] -> Logical Operator83/1
  [Con_AbsEsp_Ready2Idle] -> Logical Operator83/6
  [Con_HandOff_Ready2Idle] -> Logical Operator83/5
  [Con_YawRate_Ready2Idle] -> Logical Operator83/2
  [IP_V_Disp_kmh] -> Compare To Constant147/1
  Compare To Constant147/1 -> Logical Operator83/3  "VSM_LCK_Con_TJAVehicleSpd_Ready2Idle"
  Logical Operator83/1 -> TJA_Ready2Idle/1  "VSM_LCK_TJAReady2Idle"
  [Con_LaneCurve_Ready2Idle] -> Logical Operator83/7
  [Con_TJALane_Ready2Idle] -> Logical Operator83/4
  [TJA_Sts] -> Compare To Constant113/1, Compare To Constant115/1, Compare To Constant150/1
  Compare To Constant115/1 -> Logical Operator37/2
  Compare To Constant113/1 -> Logical Operator37/1
  [TJA_Sts] -> Compare To Constant125/1, Compare To Constant153/1, Compare To Constant126/1
  Compare To Constant125/1 -> Logical Operator39/1
  Compare To Constant126/1 -> Logical Operator39/2
  [TJA_Active] -> Switch/2
  Constant1/1 -> Switch/1
  Compare To Constant140/1 -> Logical Operator55/2
  Compare To Constant138/1 -> Logical Operator55/1
  Compare To Constant137/1 -> Logical Operator46/1
  Logical Operator55/1 -> Logical Operator59/2
  MATLAB Function1/1(y) -> Compare To Constant107/1, Compare To Constant20/1, Unit Delay4/1, Compare To Constant138/1, Compare To Constant141/1
  Logical Operator60/1 -> Goto20/1  "VSM_LCK_Con_TJAHandson_Idle2Ready"
  param_22/1 -> Compare To Constant135/1
  HandsOn1/1 -> Compare To Constant137/1
  Logical Operator59/1 -> Logical Operator60/2
  Compare To Constant135/1 -> Logical Operator60/1
  Logical Operator46/1 -> Logical Operator59/1
  Compare To Constant141/1 -> Logical Operator46/2
  From80/1 -> Compare To Constant140/1
  TJALCKState/1 -> [TJALCKState]
  LSSSwtReq/1 -> [LSSSwtReq]
  [LSSSwtReq] -> Logical Operator61/1
  [LCK_On] -> Logical Operator61/2
  [Con_DriverInput_Active2Ready] -> LCK_Con_DriverInput_ LCKExit/1  "LCK_Con_DriverInput_ LCKExit"
  [Con_AccPedalRate_Active2Ready] -> LCK_Con_AccPedalRate_LCKExit/1  "LCK_Con_AccPedalRate_LCKExit"
  [Con_BrakePress_Active2Ready] -> LCK_Con_BrakePress_ LCKExit/1  "LCK_Con_BrakePress_ LCKExit"
  [Con_OverRide_Active2Ready] -> LCK_Con_OverRide_ LCKExit/1  "LCK_Con_OverRide_ LCKExit"
  [Con_SteerWheelAngle_Active2Ready] -> LCK_Con_SteerWheelAngle_ LCKExit/1  "LCK_Con_SteerWheelAngle_ LCKExit"
  [Con_SteerAngleSpd_Active2Ready] -> LCK_Con_SteerAngleSpd_ LCKExit/1  "LCK_Con_SteerAngleSpd_ LCKExit"
  Compare To Constant150/1 -> Logical Operator37/3
  Compare To Constant153/1 -> Logical Operator39/3
  Compare To Constant43/1 -> Subsystem2/1(In1)
  Subsystem2/1(Out1) -> Compare To Constant42/1
  Compare To Constant42/1 -> Logical Operator75/3
  [LCK_Sts] -> Compare To Constant43/1
  [TJA_Active] -> Compare To Constant67/1
  Compare To Constant67/1 -> Logical Operator111/2
  [TJA_Active] -> Compare To Constant193/1
  Compare To Constant193/1 -> Logical Operator68/3
  [TJA_Active] -> Compare To Constant194/1
  Compare To Constant194/1 -> Logical Operator70/3
  [TJA_Active] -> Compare To Constant195/1
  Compare To Constant195/1 -> Logical Operator97/3
  Compare To Constant226/1 -> Logical Operator48/3
  [TJA_Active] -> Compare To Constant226/1
  [TJA_Active] -> Compare To Constant227/1
  Compare To Constant227/1 -> Logical Operator51/3
  [TJA_Active] -> Compare To Constant230/1
  Compare To Constant230/1 -> Logical Operator92/3
  [TJA_Active] -> Compare To Constant231/1
  Compare To Constant231/1 -> Logical Operator79/3
  [TJA_Active] -> Compare To Constant233/1
  Compare To Constant233/1 -> Logical Operator104/3
  [TJA_Active] -> Compare To Constant234/1
  Compare To Constant234/1 -> Logical Operator58/3
  Compare To Constant235/1 -> Logical Operator60/3
  From128/1 -> Compare To Constant235/1
  Subsystem3/1(Out1) -> Compare To Constant10/1
  Logical Operator26/1 -> Subsystem3/1(In1)
  Compare To Constant10/1 -> Logical Operator76/1
  Logical Operator76/1 -> [TJALineValid]
  [AccrPel] -> Compare To Constant40/1
  Compare To Constant40/1 -> Logical Operator77/1
  Logical Operator77/1 -> Logical Operator47/2
  Compare To Constant84/1 -> Subsystem4/1(In1)
  Subsystem4/1(Out1) -> Compare To Constant136/1
  Compare To Constant136/1 -> Logical Operator77/2
  [HWA_Sts] -> Compare To Constant210/1, Compare To Constant139/1
  Compare To Constant139/1 -> Logical Operator78/1
  Compare To Constant210/1 -> Logical Operator78/2
  Logical Operator78/1 -> Switch2/2
  Compare To Constant7/1 -> Switch2/3  "Override"
  Switch2/1 -> [OverRide], Logical Operator100/2
  Compare To Constant214/1 -> Logical Operator80/1
  Abs9/1 -> Compare To Constant214/1
  Product1/1 -> Compare To Constant213/1
  Compare To Constant213/1 -> Logical Operator80/2
  LKATrqOvlCmdReqValue1/1 -> Product1/2  "Override"
  EPS_DrvInputTrqValue1/1 -> Abs9/1, Product1/1
  Logical Operator80/1 -> Subsystem10/1(In1)
  Subsystem10/1(Out1) -> Compare To Constant237/1
  Compare To Constant237/1 -> Switch2/1  "Override"
  Compare To Constant239/1 -> Logical Operator102/2
  Compare To Constant238/1 -> Logical Operator102/1
  [HWA_Sts] -> Compare To Constant238/1, Compare To Constant239/1
  Logical Operator102/1 -> Switch3/2
  Compare To Constant91/1 -> Switch3/3
  EPS_DrvInputTrqValue4/1 -> Abs10/1
  Abs10/1 -> Compare To Constant249/1
  Compare To Constant249/1 -> Switch3/1
  Switch3/1 -> Logical Operator49/2
  Compare To Constant13/1 -> Subsystem12/1(In1)
  NOH_Sts/1 -> [NOH_Sts]
  LSM_PilotRoadSts/1 -> [LSM_PilotRoadSts]
  [NOH_Sts] -> Compare To Constant108/1
  Compare To Constant108/1 -> Switch7/1
  [NOH_Sts] -> Compare To Constant109/1
  Compare To Constant109/1 -> Switch8/1
  Constant2/1 -> Switch7/2
  Constant3/1 -> Switch8/2
  [LSM_PilotRoadSts] -> Compare To Constant143/1, Compare To Constant142/1, Compare To Constant134/1, Compare To Constant133/1, Compare To Constant132/1, Compare To Constant112/1, Compare To Constant110/1
  Compare To Constant112/1 -> Logical Operator9/2
  Compare To Constant134/1 -> Logical Operator9/5
  Compare To Constant110/1 -> Logical Operator9/1
  Compare To Constant132/1 -> Logical Operator9/3
  Compare To Constant133/1 -> Logical Operator9/4
  Compare To Constant142/1 -> Logical Operator9/6
  Compare To Constant143/1 -> Logical Operator9/7
  Compare To Constant144/1 -> Logical Operator10/2
  [NOH_Sts] -> Compare To Constant144/1
  Logical Operator10/1 -> [NOH_ExitEn], Switch7/3
  Logical Operator9/1 -> Logical Operator10/1
  Switch7/1 -> Logical Operator35/6
  [NOH_ExitEn] -> NOT1/1
  NOT1/1 -> Switch8/3
  Switch8/1 -> Logical Operator32/6
  [Con_LSMLine_Idle2Ready] -> Logical Operator12/8
  [Con_TurnLight_Ready2Active] -> Logical Operator16/1
  [Con_SteerAngleSpd_Ready2Active] -> Logical Operator16/2
  [Con_BrakePress_Ready2Active] -> Logical Operator16/3
  [Con_AccPedalRate_Ready2active] -> Logical Operator16/4
  [Con_SteerWheelAngle_Ready2active] -> Logical Operator16/5
  [Con_DrvInputTrqValue_Ready2active] -> Logical Operator16/6
  [Con_LateralAcc_Ready2Active] -> Logical Operator16/7
  [Con_LongitudeAcc_Ready2Active] -> Logical Operator16/8
  [Con_CURRENT_GEAR_Ready2Active] -> Logical Operator16/9
  [Con_OverRide_Ready2Active] -> Logical Operator16/10
  [Con_EpsSts_Ready2Active] -> Logical Operator16/11
  [Con_LaneChange_Ready2Active] -> Logical Operator16/12
  Logical Operator16/1 -> LCK_TJAReady2Active/1  "VSM_LCK_TJAReady2Active"
  [Con_TargetLaneIn_Idle2Ready] -> Logical Operator16/13
